simulink model "Simulator_hquad_lqri"  (Simulink 7.6)
settings: Solver=ode3  StartTime=0.0  StopTime=40  FixedStep=Ts  RelTol=1e-3
values from neighbouring files (symbols this model uses):
  g = 9.8065    [kostas_malakies.mat]    (also in kostas_malakies2.mat; load_PMModel.m = 9.81; main.m; main_last.m)
  mass = 0.66    [kostas_malakies.mat]    (also in kostas_malakies2.mat; load_PMModel.m = 0.687; main_last.m)
  Ts = 0.02    [kostas_malakies.mat]    (also in kostas_malakies2.mat; main.m; main_last.m; matlab.mat = 0.08)
  Ts_slow = 0.02    [kostas_malakies.mat]    (also in kostas_malakies2.mat; main.m; main_last.m)
libraries: simulink x12, Hquad_control_LIB_LQRI x11, sdolib x4, Hqaud_model_LIB_SI x1
settings Model: Creator=andi  LastModifiedBy=burrimi
settings DebuggingCC: InheritedTsInSrcMsg=none  StrictBusMsg=Warning
settings SFSimCC: SimParseCustomCode=off

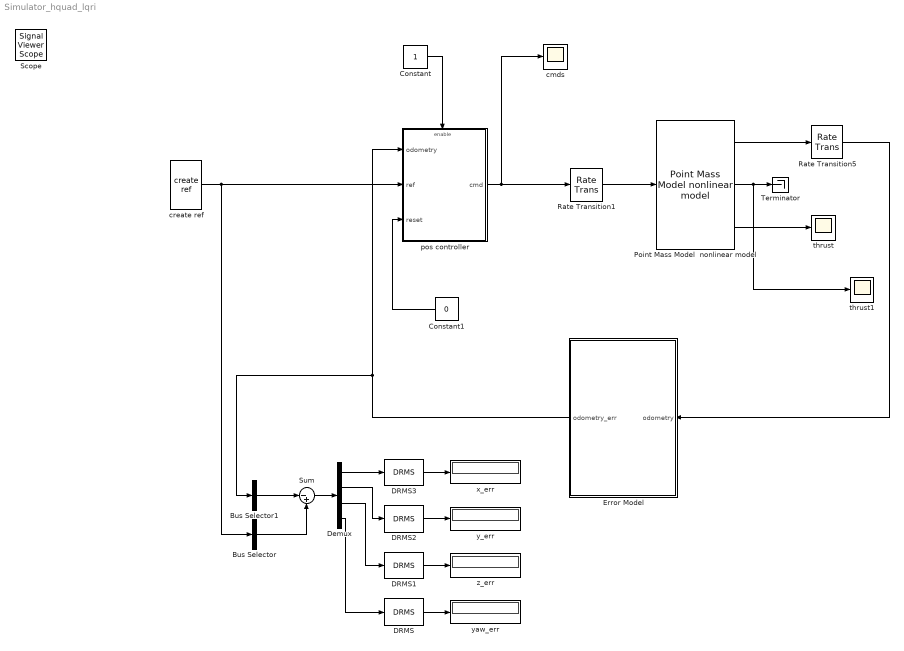
== system Simulator_hquad_lqri ==
  Bus Selector : BusSelector  OutputSignals=pose_ref.x_ref,pose_ref.y_ref,pose_ref.z_ref,pose_ref.yaw_ref  OutputAsBus=on
  Bus Selector1 : BusSelector  OutputSignals=pos.x,pos.y,pos.z,rpy.yaw  OutputAsBus=on
  Constant : Constant
  Constant1 : Constant  Value=0
  DRMS{,1..3} (4 alike) : sdolib/RMS Blocks/DRMS  SystemSampleTime=-1  Ts=Ts
  Demux : Demux
  Error Model : Subsystem
  Point Mass Model  nonlinear model : Hqaud_model_LIB_SI/Point Mass Model  nonlinear model  SystemSampleTime=-1
      link override Integrator: InitialCondition=0
      link override Integrator2: InitialCondition=0
  Rate Transition1 : RateTransition  OutPortSampleTime=Ts
  Rate Transition5 : RateTransition  OutPortSampleTime=Ts
  Sum : Sum  Inputs=|-+
  Terminator : Terminator
  cmds : Scope
      settings: TimeRange=40  YMin=-0.5  YMax=0.5
  create ref : Hquad_control_LIB_LQRI/create ref  SystemSampleTime=-1
  pos controller : Subsystem  AncestorBlock=Hquad_control_LIB_LQRI/pos controller
  thrust : Scope
      settings: TimeRange=40  YMin=113.9130434782609  YMax=138.2608695652174  SaveName=ScopeData8
  thrust1 : Scope
      settings: TimeRange=40  YMin=-2  YMax=6  SaveName=ScopeData9
  x_err : Display
  y_err : Display
  yaw_err : Display
  z_err : Display
  Scope : SignalViewerScope  IOType=viewer  LegendLocations="321.25       180.625         123.5       128.125"  RefreshTime=0.035000
      settings: ShowLegends=on
  wires:
  Point Mass Model  nonlinear model/3 -> thrust/1
  pos controller/1(cmd) -> cmds/1, Rate Transition1/1
  Constant/1 -> pos controller/Enable
  Point Mass Model  nonlinear model/2 -> Terminator/1, thrust1/1
  Constant1/1 -> pos controller/3(reset)
  create ref/1 -> Bus Selector/1, pos controller/2(ref)
  Point Mass Model  nonlinear model/1 -> Rate Transition5/1
  Error Model/1(odometry_err) -> Bus Selector1/1, pos controller/1(odometry)
  Rate Transition5/1 -> Error Model/1(odometry)
  Bus Selector1/1 -> Sum/1
  Bus Selector/1 -> Sum/2
  Sum/1 -> Demux/1
  Demux/1 -> DRMS3/1
  Demux/2 -> DRMS2/1
  Demux/3 -> DRMS1/1
  Demux/4 -> DRMS/1
  DRMS/1 -> yaw_err/1
  DRMS1/1 -> z_err/1
  DRMS2/1 -> y_err/1
  DRMS3/1 -> x_err/1
  Rate Transition1/1 -> Point Mass Model  nonlinear model/1

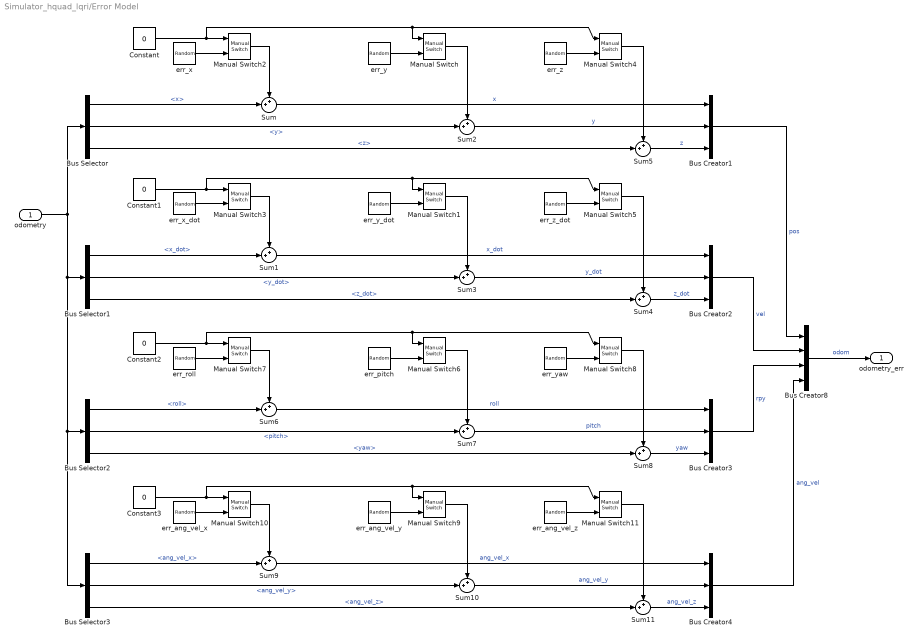
== system Simulator_hquad_lqri/Error Model ==
  odometry : Inport
  Bus Creator{1..4} (4 alike) : BusCreator  Inputs=3
  Bus Creator8 : BusCreator
  Bus Selector : BusSelector  OutputSignals=pos.x,pos.y,pos.z
  Bus Selector1 : BusSelector  OutputSignals=vel.x_dot,vel.y_dot,vel.z_dot
  Bus Selector2 : BusSelector  OutputSignals=rpy.roll,rpy.pitch,rpy.yaw
  Bus Selector3 : BusSelector  OutputSignals=ang_vel.ang_vel_x,ang_vel.ang_vel_y,ang_vel.ang_vel_z
  Constant{,1..3} (4 alike) : Constant  Value=0
  Manual Switch{,1..11} (12 alike) : simulink/Signal Routing/Manual Switch  SystemSampleTime=-1  sw=1  action=0  varsize=off
  Sum{,1..11} (12 alike) : Sum  Inputs=++|  SampleTime=Ts_slow
  err_ang_vel_x : RandomNumber  Variance=0.0001  SampleTime=Ts_slow
  err_ang_vel_y : RandomNumber  Variance=0.0001  SampleTime=Ts_slow
  err_ang_vel_z : RandomNumber  Variance=0.0001  SampleTime=Ts_slow
  err_pitch : RandomNumber  Variance=0.0001  SampleTime=Ts_slow
  err_roll : RandomNumber  Variance=0.0001  SampleTime=Ts_slow
  err_x : RandomNumber  Variance=0.000707  SampleTime=Ts_slow
  err_x_dot : RandomNumber  Variance=0.0001  SampleTime=Ts_slow
  err_y : RandomNumber  Variance=0.000707  SampleTime=Ts_slow
  err_y_dot : RandomNumber  Variance=0.0001  SampleTime=Ts_slow
  err_yaw : RandomNumber  Variance=0.0001  SampleTime=Ts_slow
  err_z : RandomNumber  Variance=0.000707  SampleTime=Ts_slow
  err_z_dot : RandomNumber  Variance=0.0001  SampleTime=Ts_slow
  odometry_err : Outport
  wires:
  err_z/1 -> Manual Switch4/2
  Manual Switch4/1 -> Sum5/1
  err_y/1 -> Manual Switch/2
  Manual Switch/1 -> Sum2/1
  err_x/1 -> Manual Switch2/2
  Manual Switch2/1 -> Sum/1
  Sum/1 -> Bus Creator1/1  "x"
  Bus Creator1/1 -> Bus Creator8/1  "pos"
  Sum2/1 -> Bus Creator1/2  "y"
  Sum5/1 -> Bus Creator1/3  "z"
  odometry/1 -> Bus Selector/1, Bus Selector2/1, Bus Selector3/1, Bus Selector1/1
  Bus Selector/1 -> Sum/2  "<x>"
  Bus Selector/2 -> Sum2/2  "<y>"
  Bus Selector/3 -> Sum5/2  "<z>"
  Constant/1 -> Manual Switch2/1, Manual Switch/1, Manual Switch4/1
  err_z_dot/1 -> Manual Switch5/2
  Manual Switch5/1 -> Sum4/1
  err_y_dot/1 -> Manual Switch1/2
  Manual Switch1/1 -> Sum3/1
  err_x_dot/1 -> Manual Switch3/2
  Manual Switch3/1 -> Sum1/1
  Sum1/1 -> Bus Creator2/1  "x_dot"
  Sum3/1 -> Bus Creator2/2  "y_dot"
  Sum4/1 -> Bus Creator2/3  "z_dot"
  Bus Selector1/1 -> Sum1/2  "<x_dot>"
  Bus Selector1/2 -> Sum3/2  "<y_dot>"
  Bus Selector1/3 -> Sum4/2  "<z_dot>"
  Constant1/1 -> Manual Switch3/1, Manual Switch1/1, Manual Switch5/1
  Bus Creator2/1 -> Bus Creator8/2  "vel"
  err_yaw/1 -> Manual Switch8/2
  Manual Switch8/1 -> Sum8/1
  err_pitch/1 -> Manual Switch6/2
  Manual Switch6/1 -> Sum7/1
  err_roll/1 -> Manual Switch7/2
  Manual Switch7/1 -> Sum6/1
  Sum6/1 -> Bus Creator3/1  "roll"
  Sum7/1 -> Bus Creator3/2  "pitch"
  Sum8/1 -> Bus Creator3/3  "yaw"
  Bus Selector2/1 -> Sum6/2  "<roll>"
  Bus Selector2/2 -> Sum7/2  "<pitch>"
  Bus Selector2/3 -> Sum8/2  "<yaw>"
  Constant2/1 -> Manual Switch7/1, Manual Switch6/1, Manual Switch8/1
  Bus Creator3/1 -> Bus Creator8/3  "rpy"
  err_ang_vel_z/1 -> Manual Switch11/2
  Manual Switch11/1 -> Sum11/1
  err_ang_vel_y/1 -> Manual Switch9/2
  Manual Switch9/1 -> Sum10/1
  err_ang_vel_x/1 -> Manual Switch10/2
  Manual Switch10/1 -> Sum9/1
  Sum9/1 -> Bus Creator4/1  "ang_vel_x"
  Sum10/1 -> Bus Creator4/2  "ang_vel_y"
  Sum11/1 -> Bus Creator4/3  "ang_vel_z"
  Bus Selector3/1 -> Sum9/2  "<ang_vel_x>"
  Bus Selector3/2 -> Sum10/2  "<ang_vel_y>"
  Bus Selector3/3 -> Sum11/2  "<ang_vel_z>"
  Constant3/1 -> Manual Switch10/1, Manual Switch9/1, Manual Switch11/1
  Bus Creator4/1 -> Bus Creator8/4  "ang_vel"
  Bus Creator8/1 -> odometry_err/1  "odom"

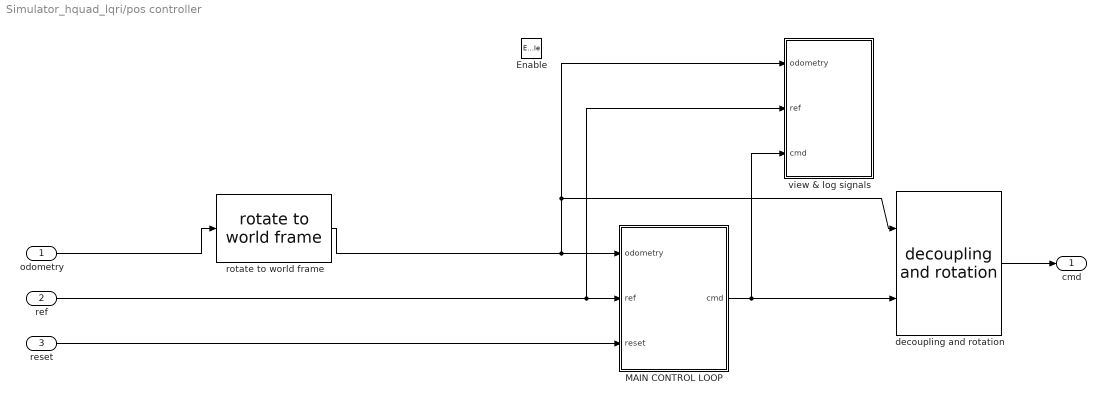
== system Simulator_hquad_lqri/pos controller ==
  odometry : Inport
  ref : Inport  Port=2
  reset : Inport  Port=3
  Enable : EnablePort  StatesWhenEnabling=reset
  MAIN CONTROL LOOP : Subsystem  AncestorBlock=Hquad_control_LIB_LQRI/MAIN CONTROL LOOP  TreatAsAtomicUnit=on
  decoupling and rotation : Hquad_control_LIB_LQRI/decoupling and rotation  Priority=3  SystemSampleTime=-1
  rotate to world frame : Hquad_control_LIB_LQRI/rotate to world frame  Priority=1  SystemSampleTime=-1
  view & log signals : Subsystem  AncestorBlock=Hquad_control_LIB_LQRI/view & log signals
  cmd : Outport
  wires:
  decoupling and rotation/1 -> cmd/1
  MAIN CONTROL LOOP/1(cmd) -> decoupling and rotation/2, view & log signals/3(cmd)
  rotate to world frame/1 -> MAIN CONTROL LOOP/1(odometry), decoupling and rotation/1, view & log signals/1(odometry)
  odometry/1 -> rotate to world frame/1
  reset/1 -> MAIN CONTROL LOOP/3(reset)
  ref/1 -> view & log signals/2(ref), MAIN CONTROL LOOP/2(ref)

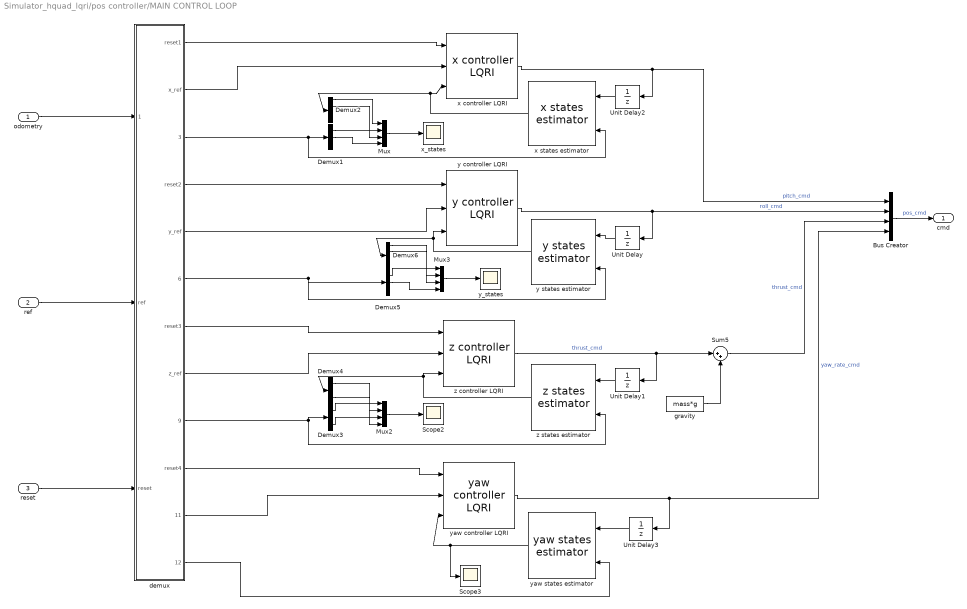
== system Simulator_hquad_lqri/pos controller/MAIN CONTROL LOOP ==
  odometry : Inport
  ref : Inport  Port=2
  reset : Inport  Port=3
  Bus Creator : BusCreator
  Demux1 : Demux  Outputs=3
  Demux2 : Demux
  Demux3 : Demux  Outputs=2
  Demux4 : Demux  Outputs=2
  Demux5 : Demux  Outputs=3
  Demux6 : Demux
  Mux : Mux
  Mux2 : Mux
  Mux3 : Mux
  Scope2 : Scope
      settings: YMin=-0.4  YMax=1.4  SaveName=ScopeData15
  Scope3 : Scope
      settings: YMin=-0.4  YMax=1.4  SaveName=ScopeData16
  Sum5 : Sum  Inputs=|++
  Unit Delay{,1..3} (4 alike) : UnitDelay  SampleTime=Ts
  demux : Subsystem
  gravity : Constant  Value=mass*g
  "x controller LQRI  " : Hquad_control_LIB_LQRI/x controller LQRI    SystemSampleTime=-1
  x states estimator : Hquad_control_LIB_LQRI/x states estimator  SystemSampleTime=-1
  x_states : Scope
      settings: TimeRange=40  YMin=-15  YMax=15  SaveName=ScopeData13
  y controller LQRI : Hquad_control_LIB_LQRI/y controller LQRI  SystemSampleTime=-1
  y states estimator : Hquad_control_LIB_LQRI/y states estimator  SystemSampleTime=-1
  y_states : Scope
      settings: TimeRange=40  YMin=-15  YMax=15  SaveName=ScopeData4
  yaw controller LQRI : Hquad_control_LIB_LQRI/yaw controller LQRI  SystemSampleTime=-1
  yaw states estimator : Hquad_control_LIB_LQRI/yaw states estimator  SystemSampleTime=-1
  z controller LQRI : Hquad_control_LIB_LQRI/z controller LQRI  SystemSampleTime=-1
  z states estimator : Hquad_control_LIB_LQRI/z states estimator  SystemSampleTime=-1
  cmd : Outport
  wires:
  Unit Delay3/1 -> yaw states estimator/1
  Sum5/1 -> Bus Creator/3  "thrust_cmd"
  demux/11(yaw_ref) -> yaw controller LQRI/2
  demux/9(z_states_meas) -> z states estimator/2, Demux3/1
  demux/6(y_states_meas) -> y states estimator/2, Demux5/1
  demux/3(x_states_meas) -> x states estimator/2, Demux1/1
  Bus Creator/1 -> cmd/1  "pos_cmd"
  demux/10(reset4) -> yaw controller LQRI/1
  demux/1(reset1) -> "x controller LQRI  "/1
  reset/1 -> demux/3(reset)
  ref/1 -> demux/2(ref)
  odometry/1 -> demux/1(odometry)
  yaw controller LQRI/1 -> Unit Delay3/1, Bus Creator/4  "yaw_rate_cmd"
  demux/12(yaw_states_meas) -> yaw states estimator/2
  Unit Delay2/1 -> x states estimator/1
  Unit Delay1/1 -> z states estimator/1
  Unit Delay/1 -> y states estimator/1
  demux/2(x_ref) -> "x controller LQRI  "/2
  x states estimator/1 -> "x controller LQRI  "/3, Demux2/1
  y states estimator/1 -> y controller LQRI/3, Demux6/1
  "x controller LQRI  "/1 -> Unit Delay2/1, Bus Creator/1  "pitch_cmd"
  y controller LQRI/1 -> Unit Delay/1, Bus Creator/2  "roll_cmd"
  z states estimator/1 -> z controller LQRI/3, Demux4/1
  Mux/1 -> x_states/1
  Mux2/1 -> Scope2/1
  Demux3/1 -> Mux2/1
  Demux4/1 -> Mux2/2
  Demux3/2 -> Mux2/3
  z controller LQRI/1 -> Unit Delay1/1, Sum5/1  "thrust_cmd"
  yaw states estimator/1 -> yaw controller LQRI/3, Scope3/1
  gravity/1 -> Sum5/2
  demux/5(y_ref) -> y controller LQRI/2
  demux/4(reset2) -> y controller LQRI/1
  Mux3/1 -> y_states/1
  Demux5/1 -> Mux3/1
  Demux6/1 -> Mux3/2
  Demux4/2 -> Mux2/4
  demux/8(z_ref) -> z controller LQRI/2
  demux/7(reset3) -> z controller LQRI/1
  Demux2/1 -> Mux/1
  Demux1/1 -> Mux/2
  Demux2/2 -> Mux/3
  Demux1/2 -> Mux/4
  Demux6/2 -> Mux3/3
  Demux5/2 -> Mux3/4

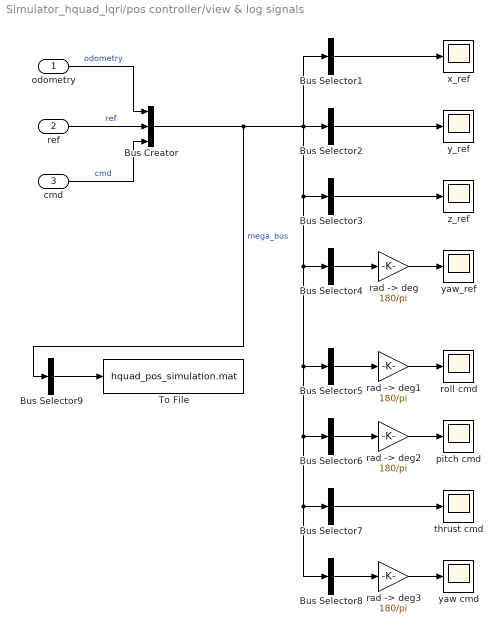
== system Simulator_hquad_lqri/pos controller/view & log signals ==
  odometry : Inport
  ref : Inport  Port=2
  cmd : Inport  Port=3
  Bus Creator : BusCreator  Inputs=3
  Bus Selector1 : BusSelector  OutputSignals=odometry.pos.x,odometry.vel.x_dot,ref.pose_ref.x_ref,ref.vel_ref.x_dot_ref  OutputAsBus=on
  Bus Selector2 : BusSelector  OutputSignals=odometry.pos.y,odometry.vel.y_dot,ref.pose_ref.y_ref,ref.vel_ref.y_dot_ref  OutputAsBus=on
  Bus Selector3 : BusSelector  OutputSignals=odometry.pos.z,odometry.vel.z_dot,ref.pose_ref.z_ref,ref.vel_ref.z_dot_ref  OutputAsBus=on
  Bus Selector4 : BusSelector  OutputSignals=odometry.rpy.yaw,odometry.ang_vel.ang_vel_z,ref.pose_ref.yaw_ref,ref.vel_ref.yaw_dot_ref  OutputAsBus=on
  Bus Selector5 : BusSelector  OutputSignals=odometry.rpy.roll,odometry.ang_vel.ang_vel_x,cmd.roll_cmd  OutputAsBus=on
  Bus Selector6 : BusSelector  OutputSignals=odometry.rpy.pitch,odometry.ang_vel.ang_vel_y,cmd.pitch_cmd  OutputAsBus=on
  Bus Selector7 : BusSelector  OutputSignals=odometry.pos.z,ref.pose_ref.z_ref,cmd.thrust_cmd  OutputAsBus=on
  Bus Selector8 : BusSelector  OutputSignals=odometry.rpy.yaw,odometry.ang_vel.ang_vel_z,cmd.yaw_rate_cmd  OutputAsBus=on
  Bus Selector9 : BusSelector  OutputSignals=odometry.pos.x,odometry.vel.x_dot,odometry.rpy.pitch,ref.pose_ref.x_ref,cmd.pitch_cmd,odometry.pos.y,odometry.vel.y_dot,odometry.rpy.roll,ref.pose_ref.y_ref,cmd.roll_cmd,odometry.pos.z,odometry.vel.z_dot,ref.pose_ref.z_ref,cmd.thrust_cmd,odometry.rpy.yaw,odometry.ang_vel.ang_vel_z,ref.pose_ref.yaw_ref,cmd.yaw_rate_cmd  OutputAsBus=on
  To File : ToFile  Filename=hquad_pos_simulation.mat  MatrixName=hquad_pos_simulation
  pitch cmd : Scope
      settings: YMin=-15  YMax=15  SaveName=ScopeData2
  rad -> deg{,1..3} (4 alike) : Gain  Gain=180/pi
  roll cmd : Scope
      settings: YMin=-100  YMax=100
  thrust cmd : Scope
      settings: YMin=-3  YMax=3  SaveName=ScopeData11
  x_ref : Scope
      settings: TimeRange=40  YMin=-0.3  YMax=1.3  SaveName=ScopeData3
  y_ref : Scope
      settings: TimeRange=40  YMin=-1.5  YMax=1.5
  yaw cmd : Scope
      settings: YMin=-60  YMax=-0  SaveName=ScopeData10
  yaw_ref : Scope
      settings: TimeRange=39.996  YMin=0  YMax=3250  SaveName=ScopeData8
  z_ref : Scope
      settings: YMin=-0.05  YMax=1.05  SaveName=ScopeData5
  wires:
  Bus Selector8/1 -> "rad -> deg3"/1
  Bus Selector6/1 -> "rad -> deg2"/1
  Bus Selector5/1 -> "rad -> deg1"/1
  Bus Selector7/1 -> thrust cmd/1
  Bus Selector4/1 -> "rad -> deg"/1
  Bus Selector3/1 -> z_ref/1
  Bus Selector2/1 -> y_ref/1
  Bus Selector1/1 -> x_ref/1
  Bus Creator/1 -> Bus Selector8/1, Bus Selector7/1, Bus Selector6/1, Bus Selector5/1, Bus Selector4/1, Bus Selector3/1, Bus Selector2/1, Bus Selector1/1, Bus Selector9/1  "mega_bus"
  cmd/1 -> Bus Creator/3  "cmd"
  ref/1 -> Bus Creator/2  "ref"
  odometry/1 -> Bus Creator/1  "odometry"
  "rad -> deg3"/1 -> yaw cmd/1
  "rad -> deg2"/1 -> pitch cmd/1
  "rad -> deg1"/1 -> roll cmd/1
  "rad -> deg"/1 -> yaw_ref/1
  Bus Selector9/1 -> To File/1

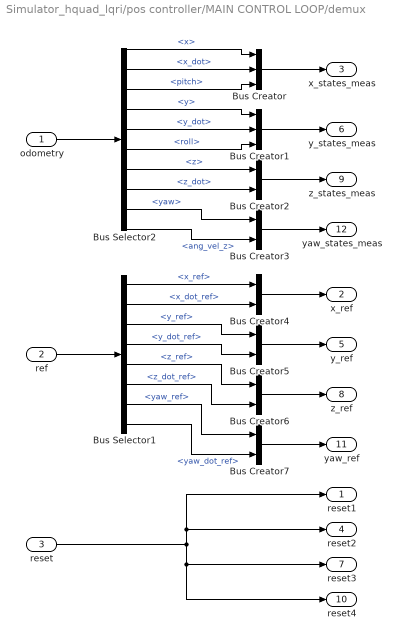
== system Simulator_hquad_lqri/pos controller/MAIN CONTROL LOOP/demux ==
  odometry : Inport
  ref : Inport  Port=2
  reset : Inport  Port=3
  Bus Creator : BusCreator  Inputs=3
  Bus Creator1 : BusCreator  Inputs=3
  Bus Creator{2..7} (6 alike) : BusCreator  Inputs=2
  Bus Selector1 : BusSelector  OutputSignals=pose_ref.x_ref,vel_ref.x_dot_ref,pose_ref.y_ref,vel_ref.y_dot_ref,pose_ref.z_ref,vel_ref.z_dot_ref,pose_ref.yaw_ref,vel_ref.yaw_dot_ref
  Bus Selector2 : BusSelector  OutputSignals=pos.x,vel.x_dot,rpy.pitch,pos.y,vel.y_dot,rpy.roll,pos.z,vel.z_dot,rpy.yaw,ang_vel.ang_vel_z
  reset1 : Outport
  x_ref : Outport  Port=2  PortDimensions=2
  x_states_meas : Outport  Port=3  PortDimensions=3
  reset2 : Outport  Port=4
  y_ref : Outport  Port=5  PortDimensions=2
  y_states_meas : Outport  Port=6  PortDimensions=3
  reset3 : Outport  Port=7
  z_ref : Outport  Port=8  PortDimensions=2
  z_states_meas : Outport  Port=9  PortDimensions=2
  reset4 : Outport  Port=10
  yaw_ref : Outport  Port=11  PortDimensions=2
  yaw_states_meas : Outport  Port=12  PortDimensions=2
  wires:
  reset/1 -> reset1/1, reset2/1, reset4/1, reset3/1
  Bus Selector1/8 -> Bus Creator7/2  "<yaw_dot_ref>"
  Bus Selector1/7 -> Bus Creator7/1  "<yaw_ref>"
  Bus Selector1/6 -> Bus Creator6/2  "<z_dot_ref>"
  Bus Selector1/5 -> Bus Creator6/1  "<z_ref>"
  Bus Selector1/4 -> Bus Creator5/2  "<y_dot_ref>"
  Bus Selector1/3 -> Bus Creator5/1  "<y_ref>"
  Bus Selector1/2 -> Bus Creator4/2  "<x_dot_ref>"
  Bus Creator4/1 -> x_ref/1
  Bus Creator5/1 -> y_ref/1
  Bus Creator6/1 -> z_ref/1
  Bus Creator7/1 -> yaw_ref/1
  Bus Selector1/1 -> Bus Creator4/1  "<x_ref>"
  ref/1 -> Bus Selector1/1
  Bus Creator3/1 -> yaw_states_meas/1
  Bus Creator2/1 -> z_states_meas/1
  Bus Selector2/10 -> Bus Creator3/2  "<ang_vel_z>"
  Bus Selector2/9 -> Bus Creator3/1  "<yaw>"
  Bus Selector2/8 -> Bus Creator2/2  "<z_dot>"
  Bus Selector2/7 -> Bus Creator2/1  "<z>"
  Bus Creator1/1 -> y_states_meas/1
  Bus Selector2/5 -> Bus Creator1/2  "<y_dot>"
  Bus Selector2/4 -> Bus Creator1/1  "<y>"
  Bus Selector2/2 -> Bus Creator/2  "<x_dot>"
  Bus Selector2/1 -> Bus Creator/1  "<x>"
  Bus Creator/1 -> x_states_meas/1
  odometry/1 -> Bus Selector2/1
  Bus Selector2/3 -> Bus Creator/3  "<pitch>"
  Bus Selector2/6 -> Bus Creator1/3  "<roll>"
